simulink model "FormulaElectricSimTool"  (R2015a)
settings: Solver=ode1  StartTime=0.0  StopTime=DriveCycle.Tf  FixedStep=Sim.TimeStep  RelTol=1e-3
undefined symbols (not defined in the file): Battery, Brake, DriveCycle, Driver, g, magnitude, Motor, Sim, Veh
libraries: AMKMotor x4, simulink x3, Battery x1
settings Model: CovSFcnEnable=off  Creator=tbria  LastModifiedBy=tbria
settings DataIOCC: LimitDataPoints=off
settings DebuggingCC: SolverPrmCheckMsg=warning

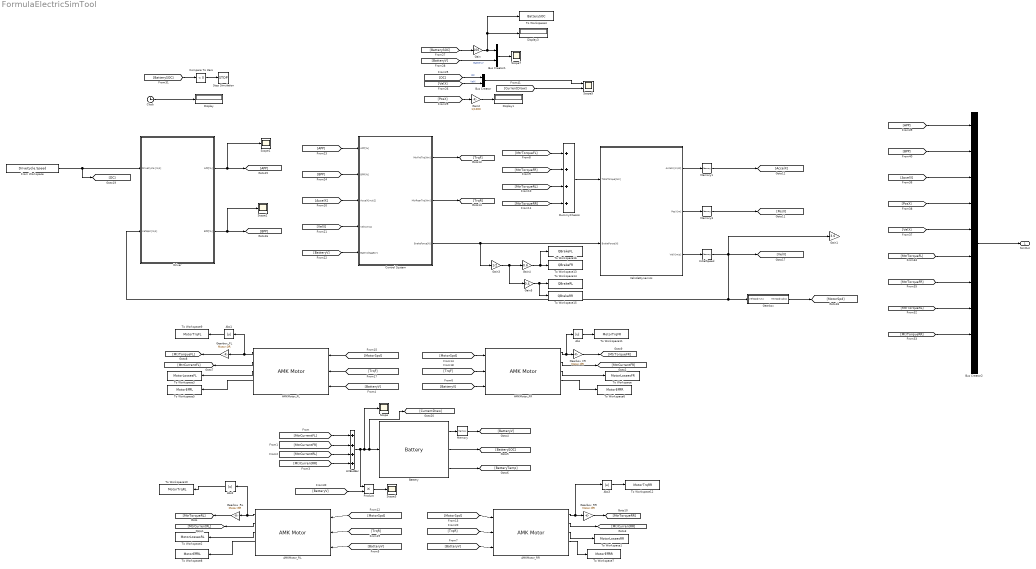
== system FormulaElectricSimTool ==
  AMKMotor_FL : AMKMotor/WheelAssembly/AMK Motor
  AMKMotor_FR : AMKMotor/WheelAssembly/AMK Motor
  AMKMotor_RL : AMKMotor/WheelAssembly/AMK Motor
  AMKMotor_RR : AMKMotor/WheelAssembly/AMK Motor
  Abs{,1..3} (4 alike) : Abs
  Battery : Battery/Battery
  Bus Creator : BusCreator  Inputs=2
  Bus Creator1 : BusCreator  Inputs=2
  Bus Creator2 : BusCreator  Inputs=10
  Clock : Clock
  Compare To Zero : simulink/Logic and Bit Operations/Compare To Zero  relop=<  OutDataTypeStr=boolean
  Control System : Subsystem
  Display : Display
  Display1 : Display
  Display3 : Display
  Driver : Subsystem
  DummyChassis : Sum  Inputs=++++
  From Workspace : FromWorkspace  VariableName=DriveCycle.Speed  SampleTime=0
  Gain : Gain  Gain=100
  Gain1 : Gain  Gain=3.6
  Gain2 : Gain  Gain=1/1000
  Gain3 : Gain  Gain=1/2
  Gain4 : Gain  Gain=0.6
  Gain5 : Gain  Gain=0.4
  Gearbox : Subsystem
  Gearbox_FL : Gain  Gain=Motor.GR
  Gearbox_FR : Gain  Gain=Motor.GR
  Gearbox_RL : Gain  Gain=Motor.GR
  Gearbox_RR : Gain  Gain=Motor.GR
  HVBusBar : Sum  Inputs=4
  InitialSpeed : Memory  X0=DriveCycle.Vi
  Memory : Memory  X0=600
  Memory1 : Memory
  Memory3 : Memory
  Product : Product
  Scope{,1..3,7} (5 alike) : Scope
      Scope2 settings: SaveName=ScopeData2
      Scope3 settings: SaveName=ScopeData3
      Scope7 settings: ShowLegends=on  SaveName=ScopeData7
  Scope5 : Scope  NumInputPorts=2
      settings: ShowLegends=on  YMin=7.5~-5  YMax=37.5~5  SaveName=ScopeData5
  Stop Simulation : Stop
  To Workspace : ToWorkspace  VariableName=MotorLossesFR  SampleTime=-1
      settings: Decimation=3  Save2DSignal=2-D array (concatenate along first dimension)
  To Workspace1 : ToWorkspace  VariableName=MotorLossesRR  SampleTime=-1
      settings: Decimation=3  Save2DSignal=2-D array (concatenate along first dimension)
  To Workspace10 : ToWorkspace  VariableName=MotorTrqRL  SampleTime=-1
      settings: Decimation=3  Save2DSignal=2-D array (concatenate along first dimension)
  To Workspace11 : ToWorkspace  VariableName=MotorTrqFR  SampleTime=-1
      settings: Decimation=3  Save2DSignal=2-D array (concatenate along first dimension)
  To Workspace12 : ToWorkspace  VariableName=MotorTrqRR  SampleTime=-1
      settings: Decimation=3  Save2DSignal=2-D array (concatenate along first dimension)
  To Workspace13 : ToWorkspace  VariableName=QBrakeFR  SampleTime=-1
      settings: Decimation=3  Save2DSignal=2-D array (concatenate along first dimension)
  To Workspace14 : ToWorkspace  VariableName=QBrakeRL  SampleTime=-1
      settings: Decimation=3  Save2DSignal=2-D array (concatenate along first dimension)
  To Workspace15 : ToWorkspace  VariableName=QBrakeRR  SampleTime=-1
      settings: Decimation=3  Save2DSignal=2-D array (concatenate along first dimension)
  To Workspace16 : ToWorkspace  VariableName=QBrakeFL  SampleTime=-1
      settings: Decimation=3  Save2DSignal=2-D array (concatenate along first dimension)
  To Workspace2 : ToWorkspace  VariableName=MotorLossesRL  SampleTime=-1
      settings: Decimation=3  Save2DSignal=2-D array (concatenate along first dimension)
  To Workspace3 : ToWorkspace  VariableName=MotorLossesFL  SampleTime=-1
      settings: Decimation=3  Save2DSignal=2-D array (concatenate along first dimension)
  To Workspace4 : ToWorkspace  VariableName=BatterySOC  SampleTime=-1
      settings: Save2DSignal=2-D array (concatenate along first dimension)
  To Workspace5 : ToWorkspace  VariableName=MotorEffFL  SaveFormat=Timeseries  SampleTime=-1
  To Workspace6 : ToWorkspace  VariableName=MotorEffFR  SaveFormat=Timeseries  SampleTime=-1
  To Workspace7 : ToWorkspace  VariableName=MotorEffRR  SaveFormat=Timeseries  SampleTime=-1
  To Workspace8 : ToWorkspace  VariableName=MotorEffRL  SaveFormat=Timeseries  SampleTime=-1
  To Workspace9 : ToWorkspace  VariableName=MotorTrqFL  SampleTime=-1
      settings: Decimation=3  Save2DSignal=2-D array (concatenate along first dimension)
  VehicleDynamics : Subsystem
  SimOut : Outport
  wires:
  HVBusBar/1 -> Product/1, Scope/1, [CurrentDraw], Battery/1
  [MtrCurrentFL] -> HVBusBar/1
  [MtrCurrentFR] -> HVBusBar/2
  [MtrCurrentRL] -> HVBusBar/3
  [MtrCurrentRR] -> HVBusBar/4
  Battery/1 -> Memory/1
  Battery/2 -> [BatterySOC]
  Battery/3 -> [BatteryTemp]
  [BatteryV] -> AMKMotor_FL/3
  [BatteryV] -> AMKMotor_RL/3
  [BatteryV] -> AMKMotor_RR/3
  AMKMotor_RR/2 -> [MtrCurrentRR]
  AMKMotor_FR/2 -> [MtrCurrentFR]
  AMKMotor_FL/2 -> [MtrCurrentFL]
  AMKMotor_RL/2 -> [MtrCurrentRL]
  [BatteryV] -> AMKMotor_FR/3
  AMKMotor_RL/1 -> Abs2/1, Gearbox_RL/1
  AMKMotor_FL/1 -> Abs1/1, Gearbox_FL/1
  AMKMotor_FR/1 -> Abs/1, Gearbox_FR/1
  AMKMotor_RR/1 -> Abs3/1, Gearbox_RR/1
  Gearbox_RL/1 -> [MtrTorqueRL]
  Gearbox_FL/1 -> [MtrTorqueFL]
  Gearbox_FR/1 -> [MtrTorqueFR]
  Gearbox_RR/1 -> [MtrTorqueRR]
  [MtrTorqueFL] -> DummyChassis/1
  [MtrTorqueFR] -> DummyChassis/2
  [MtrTorqueRL] -> DummyChassis/3
  [MtrTorqueRR] -> DummyChassis/4
  [MotorSpd] -> AMKMotor_RL/1
  [MotorSpd] -> AMKMotor_RR/1
  [MotorSpd] -> AMKMotor_FR/1
  [MotorSpd] -> AMKMotor_FL/1
  [AccelX] -> Control System/3(AccelX[m/s2])
  Control System/2(MtrRearTrq[Nm]) -> [TrqR]
  [TrqF] -> AMKMotor_FL/2
  [TrqF] -> AMKMotor_FR/2
  [TrqR] -> AMKMotor_RL/2
  [TrqR] -> AMKMotor_RR/2
  [VelX] -> Control System/4(VelX[m/s])
  [BatteryV] -> Control System/5(BattVoltage[V])
  Control System/1(MtrFntTrq[Nm]) -> [TrqF]
  Driver/1(APP[%]) -> Scope1/1, [APP]
  Driver/2(BPP[%]) -> Scope2/1, [BPP]
  [APP] -> Control System/1(APP[%])
  [BPP] -> Control System/2(BPP[%])
  DummyChassis/1 -> VehicleDynamics/1(TotalTorque[Nm])
  VehicleDynamics/1(AccelX[m/s2]) -> Memory1/1
  VehicleDynamics/2(PosX[m]) -> Memory3/1
  VehicleDynamics/3(VelX[m/s]) -> InitialSpeed/1
  Gearbox/1(MtrSpd[rad/s]) -> [MotorSpd]
  From Workspace/1 -> [DC], Driver/1(DriveCycle [m/s])
  Clock/1 -> Display/1
  Memory1/1 -> [AccelX]
  Memory/1 -> [BatteryV]
  Memory3/1 -> [PosX]
  InitialSpeed/1 -> Driver/2(VehSpd [m/s]), Gearbox/1(VehSpd[m/s]), Gain1/1, [VelX]
  [DC] -> Bus Creator/1  "DC"
  [VelX] -> Bus Creator/2  "VelX"
  Bus Creator/1 -> Scope5/1
  Control System/3(BrakeForce[N]) -> Gain3/1, VehicleDynamics/2(BrakeForce[N])
  [BatterySOC] -> Gain/1
  [BatteryV] -> Bus Creator1/2  "BatteryV"
  Bus Creator1/1 -> Scope7/1
  Gain/1 -> To Workspace4/1, Display3/1, Bus Creator1/1
  [PosX] -> Gain2/1
  [BatteryV] -> Product/2
  Product/1 -> Scope3/1
  [BatterySOC] -> Compare To Zero/1
  Compare To Zero/1 -> Stop Simulation/1
  AMKMotor_FR/3 -> To Workspace/1
  AMKMotor_RR/3 -> To Workspace1/1
  AMKMotor_RL/3 -> To Workspace2/1
  AMKMotor_FL/3 -> To Workspace3/1
  AMKMotor_FL/4 -> To Workspace5/1
  AMKMotor_FR/4 -> To Workspace6/1
  AMKMotor_RR/4 -> To Workspace7/1
  AMKMotor_RL/4 -> To Workspace8/1
  Abs/1 -> To Workspace11/1
  Abs1/1 -> To Workspace9/1
  Abs2/1 -> To Workspace10/1
  Abs3/1 -> To Workspace12/1
  Bus Creator2/1 -> SimOut/1
  [AccelX] -> Bus Creator2/3
  [APP] -> Bus Creator2/1
  [BPP] -> Bus Creator2/2
  [PosX] -> Bus Creator2/4
  [VelX] -> Bus Creator2/5
  [MtrTorqueFL] -> Bus Creator2/6
  [MtrTorqueFR] -> Bus Creator2/7
  [MtrTorqueRL] -> Bus Creator2/8
  [MtrTorqueRR] -> Bus Creator2/9
  Gain2/1 -> Display1/1
  [CurrentDraw] -> Scope5/2
  Gain3/1 -> Gain5/1, Gain4/1
  Gain4/1 -> To Workspace16/1, To Workspace13/1
  Gain5/1 -> To Workspace15/1, To Workspace14/1

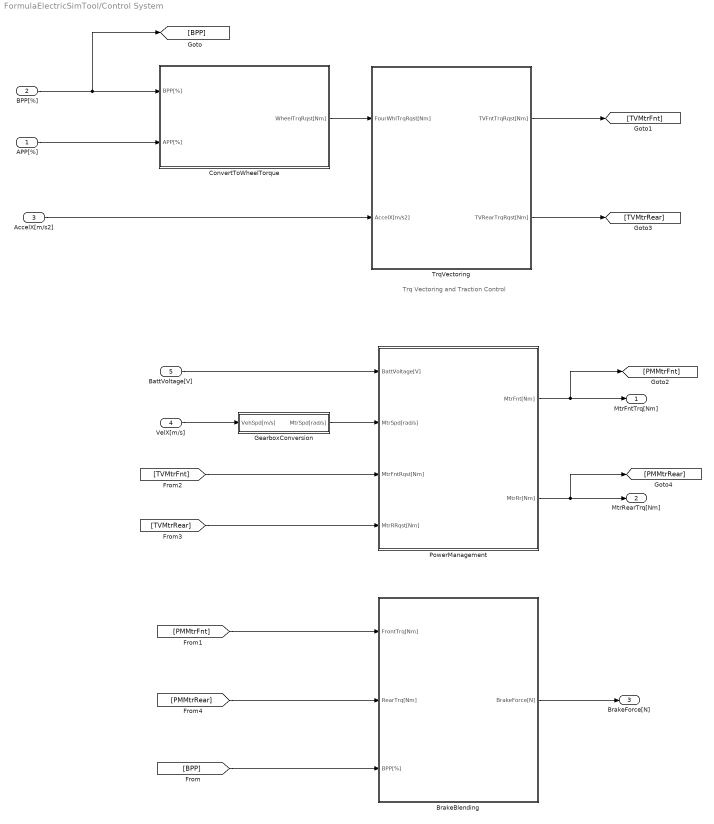
== system FormulaElectricSimTool/Control System ==
  note: Trq Vectoring and Traction Control
  APP[%] : Inport
  BPP[%] : Inport  Port=2
  AccelX[m/s2] : Inport  Port=3
  VelX[m/s] : Inport  Port=4
  BattVoltage[V] : Inport  Port=5
  BrakeBlending : Subsystem
  ConvertToWheelTorque : Subsystem
  GearboxConversion : Subsystem
  PowerManagement : Subsystem
  TrqVectoring : Subsystem
  MtrFntTrq[Nm] : Outport
  MtrRearTrq[Nm] : Outport  Port=2
  BrakeForce[N] : Outport  Port=3
  wires:
  AccelX[m/s2]/1 -> TrqVectoring/2(AccelX[m/s2])
  TrqVectoring/1(TVFntTrqRqst[Nm]) -> [TVMtrFnt]
  TrqVectoring/2(TVRearTrqRqst[Nm]) -> [TVMtrRear]
  BattVoltage[V]/1 -> PowerManagement/1(BattVoltage[V])
  [TVMtrFnt] -> PowerManagement/3(MtrFntRqst[Nm])
  [TVMtrRear] -> PowerManagement/4(MtrRRqst[Nm])
  PowerManagement/1(MtrFnt[Nm]) -> [PMMtrFnt], MtrFntTrq[Nm]/1
  PowerManagement/2(MtrRr[Nm]) -> [PMMtrRear], MtrRearTrq[Nm]/1
  VelX[m/s]/1 -> GearboxConversion/1(VehSpd[m/s])
  GearboxConversion/1(MtrSpd[rad/s]) -> PowerManagement/2(MtrSpd[rad/s])
  ConvertToWheelTorque/1(WheelTrqRqst[Nm]) -> TrqVectoring/1(FourWhlTrqRqst[Nm])
  BrakeBlending/1(BrakeForce[N]) -> BrakeForce[N]/1
  [BPP] -> BrakeBlending/3(BPP[%])
  [PMMtrFnt] -> BrakeBlending/1(FrontTrq[Nm])
  [PMMtrRear] -> BrakeBlending/2(RearTrq[Nm])
  BPP[%]/1 -> [BPP], ConvertToWheelTorque/1(BPP[%])
  APP[%]/1 -> ConvertToWheelTorque/2(APP[%])

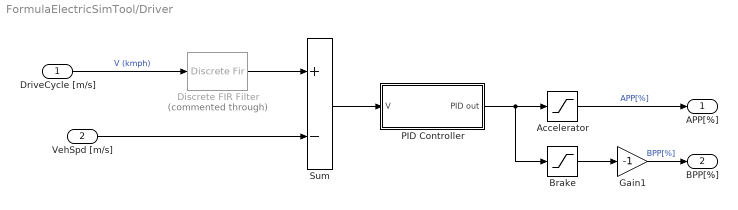
== system FormulaElectricSimTool/Driver ==
  DriveCycle [m/s] : Inport
  VehSpd [m/s] : Inport  Port=2
  Accelerator : Saturate  UpperLimit=100  LowerLimit=0
  Brake : Saturate  UpperLimit=0  LowerLimit=-100
  Discrete FIR Filter : DiscreteFir  Commented=through  Coefficients=[100:-1:0]/sum([100:-1:0])  SampleTime=Sim.TimeStep
  Gain1 : Gain  Gain=-1
  PID Controller : Subsystem
  Sum : Sum  Inputs=+-
  APP[%] : Outport
  BPP[%] : Outport  Port=2
  wires:
  VehSpd [m/s]/1 -> Sum/2
  Sum/1 -> PID Controller/1(V)
  DriveCycle [m/s]/1 -> Discrete FIR Filter/1  "V (kmph)"
  PID Controller/1("PID out ") -> Brake/1, Accelerator/1
  Accelerator/1 -> APP[%]/1  "APP[%]"
  Brake/1 -> Gain1/1
  Gain1/1 -> BPP[%]/1  "BPP[%]"
  Discrete FIR Filter/1 -> Sum/1

== system FormulaElectricSimTool/Gearbox ==
  VehSpd[m/s] : Inport
  MotorGR : Gain  Gain=Motor.GR
  WheelRadius : Gain  Gain=1/(Veh.Whl.r + Veh.Whl.SidewallH)
  MtrSpd[rad/s] : Outport
  wires:
  WheelRadius/1 -> MotorGR/1  "WhlSpd [rad/s]"
  VehSpd[m/s]/1 -> WheelRadius/1
  MotorGR/1 -> MtrSpd[rad/s]/1  "MtrSpd [rad/s]"

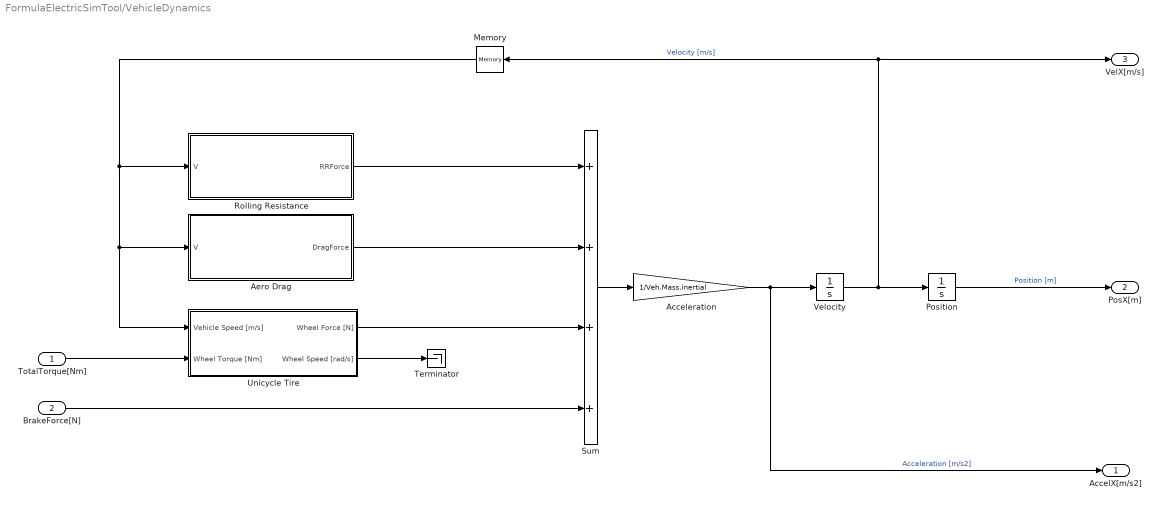
== system FormulaElectricSimTool/VehicleDynamics ==
  TotalTorque[Nm] : Inport
  BrakeForce[N] : Inport  Port=2
  Acceleration : Gain  Gain=1/Veh.Mass.inertial
  Aero Drag : Subsystem
  Memory : Memory
  Position : Integrator
  Rolling Resistance : Subsystem
  Sum : Sum  Inputs=++++
  Terminator : Terminator
  Unicycle Tire : Subsystem
  Velocity : Integrator  InitialCondition=DriveCycle.Vi
  AccelX[m/s2] : Outport
  PosX[m] : Outport  Port=2
  VelX[m/s] : Outport  Port=3
  wires:
  Memory/1 -> Unicycle Tire/1(Vehicle Speed [m/s]), Aero Drag/1(V), Rolling Resistance/1(V)
  Acceleration/1 -> AccelX[m/s2]/1, Velocity/1  "Acceleration [m/s2]"
  TotalTorque[Nm]/1 -> Unicycle Tire/2(Wheel Torque [Nm])
  Rolling Resistance/1(RRForce) -> Sum/1
  Aero Drag/1(DragForce) -> Sum/2
  Sum/1 -> Acceleration/1
  Unicycle Tire/1(Wheel Force [N]) -> Sum/3
  Unicycle Tire/2(Wheel Speed [rad/s]) -> Terminator/1
  Velocity/1 -> VelX[m/s]/1, Memory/1, Position/1  "Velocity [m/s]"
  Position/1 -> PosX[m]/1  "Position [m]"
  BrakeForce[N]/1 -> Sum/4

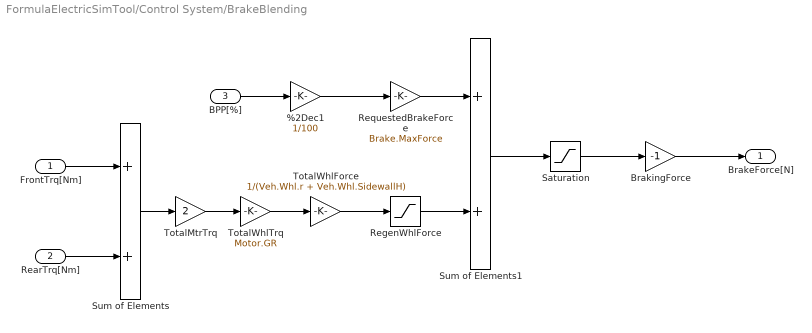
== system FormulaElectricSimTool/Control System/BrakeBlending ==
  FrontTrq[Nm] : Inport
  RearTrq[Nm] : Inport  Port=2
  BPP[%] : Inport  Port=3
  %2Dec1 : Gain  Gain=1/100
  BrakingForce : Gain  Gain=-1
  RegenWhlForce : Saturate  UpperLimit=0  LowerLimit=-inf
  RequestedBrakeForce : Gain  Gain=Brake.MaxForce
  Saturation : Saturate  UpperLimit=inf  LowerLimit=0
  Sum of Elements : Sum  Inputs=2
  Sum of Elements1 : Sum
  TotalMtrTrq : Gain  Gain=2
  TotalWhlForce : Gain  Gain=1/(Veh.Whl.r + Veh.Whl.SidewallH)
  TotalWhlTrq : Gain  Gain=Motor.GR
  BrakeForce[N] : Outport
  wires:
  FrontTrq[Nm]/1 -> Sum of Elements/1
  RearTrq[Nm]/1 -> Sum of Elements/2
  TotalMtrTrq/1 -> TotalWhlTrq/1
  %2Dec1/1 -> RequestedBrakeForce/1
  BPP[%]/1 -> %2Dec1/1
  RequestedBrakeForce/1 -> Sum of Elements1/1
  TotalWhlForce/1 -> RegenWhlForce/1
  Sum of Elements1/1 -> Saturation/1
  Saturation/1 -> BrakingForce/1
  Sum of Elements/1 -> TotalMtrTrq/1
  TotalWhlTrq/1 -> TotalWhlForce/1
  RegenWhlForce/1 -> Sum of Elements1/2
  BrakingForce/1 -> BrakeForce[N]/1

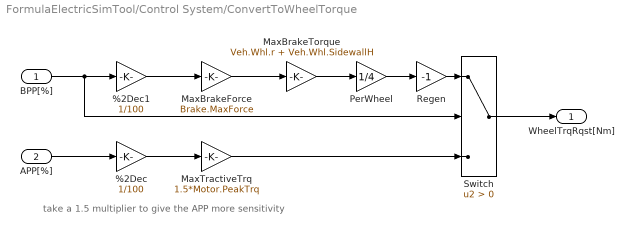
== system FormulaElectricSimTool/Control System/ConvertToWheelTorque ==
  note: take a 1.5 multiplier to give the APP more sensitivity
  BPP[%] : Inport
  APP[%] : Inport  Port=2
  %2Dec : Gain  Gain=1/100
  %2Dec1 : Gain  Gain=1/100
  MaxBrakeForce : Gain  Gain=Brake.MaxForce
  MaxBrakeTorque : Gain  Gain=Veh.Whl.r + Veh.Whl.SidewallH
  "MaxTractiveTrq " : Gain  Gain=1.5*Motor.PeakTrq
  PerWheel : Gain  Gain=1/4
  Regen : Gain  Gain=-1
  Switch : Switch  Criteria=u2 > Threshold
  WheelTrqRqst[Nm] : Outport
  wires:
  PerWheel/1 -> Regen/1
  "MaxTractiveTrq "/1 -> Switch/3
  %2Dec/1 -> "MaxTractiveTrq "/1
  MaxBrakeForce/1 -> MaxBrakeTorque/1
  MaxBrakeTorque/1 -> PerWheel/1
  BPP[%]/1 -> Switch/2, %2Dec1/1
  %2Dec1/1 -> MaxBrakeForce/1
  Switch/1 -> WheelTrqRqst[Nm]/1
  APP[%]/1 -> %2Dec/1
  Regen/1 -> Switch/1

== system FormulaElectricSimTool/Control System/GearboxConversion ==
  VehSpd[m/s] : Inport
  MotorGR : Gain  Gain=Motor.GR
  WheelRadius : Gain  Gain=1/(Veh.Whl.r + Veh.Whl.SidewallH)
  MtrSpd[rad/s] : Outport
  wires:
  WheelRadius/1 -> MotorGR/1  "WhlSpd [rad/s]"
  VehSpd[m/s]/1 -> WheelRadius/1
  MotorGR/1 -> MtrSpd[rad/s]/1  "MtrSpd [rad/s]"

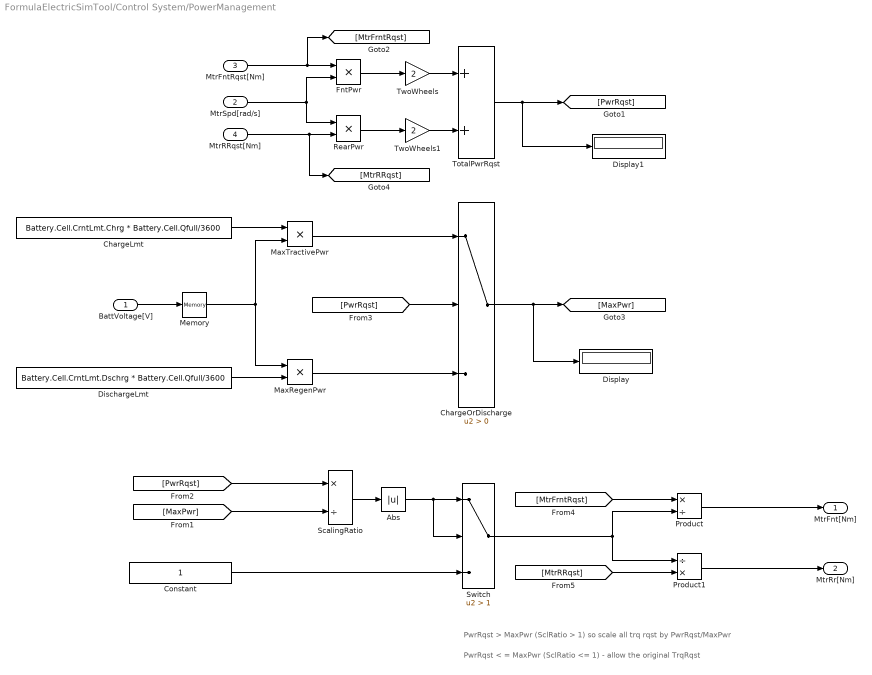
== system FormulaElectricSimTool/Control System/PowerManagement ==
  note: PwrRqst > MaxPwr (SclRatio > 1) so scale all trq rqst by PwrRqst/MaxPwr
  note: PwrRqst < = MaxPwr (SclRatio <= 1) - allow the original TrqRqst
  BattVoltage[V] : Inport
  MtrSpd[rad/s] : Inport  Port=2
  MtrFntRqst[Nm] : Inport  Port=3
  MtrRRqst[Nm] : Inport  Port=4
  Abs : Abs
  ChargeLmt : Constant  Value=Battery.Cell.CrntLmt.Chrg * Battery.Cell.Qfull/3600
  ChargeOrDischarge : Switch  Criteria=u2 > Threshold
  Constant : Constant
  DischargeLmt : Constant  Value=Battery.Cell.CrntLmt.Dschrg * Battery.Cell.Qfull/3600
  Display : Display
  Display1 : Display
  FntPwr : Product
  MaxRegenPwr : Product
  MaxTractivePwr : Product
  Memory : Memory  X0=600
  Product : Product  Inputs=*/
  Product1 : Product  Inputs=/*
  RearPwr : Product
  ScalingRatio : Product  Inputs=*/
  Switch : Switch  Criteria=u2 > Threshold  Threshold=1
  TotalPwrRqst : Sum
  TwoWheels : Gain  Gain=2
  TwoWheels1 : Gain  Gain=2
  MtrFnt[Nm] : Outport
  MtrRr[Nm] : Outport  Port=2
  wires:
  ChargeLmt/1 -> MaxTractivePwr/1
  BattVoltage[V]/1 -> Memory/1
  DischargeLmt/1 -> MaxRegenPwr/2
  MaxTractivePwr/1 -> ChargeOrDischarge/1
  MaxRegenPwr/1 -> ChargeOrDischarge/3
  ChargeOrDischarge/1 -> Display/1, [MaxPwr]
  [MaxPwr] -> ScalingRatio/2
  [PwrRqst] -> ScalingRatio/1
  ScalingRatio/1 -> Abs/1
  Abs/1 -> Switch/1, Switch/2
  MtrSpd[rad/s]/1 -> RearPwr/1, FntPwr/2
  MtrRRqst[Nm]/1 -> [MtrRRqst], RearPwr/2
  FntPwr/1 -> TwoWheels/1
  RearPwr/1 -> TwoWheels1/1
  TwoWheels1/1 -> TotalPwrRqst/2
  TotalPwrRqst/1 -> Display1/1, [PwrRqst]
  TwoWheels/1 -> TotalPwrRqst/1
  [PwrRqst] -> ChargeOrDischarge/2
  MtrFntRqst[Nm]/1 -> [MtrFrntRqst], FntPwr/1
  Switch/1 -> Product/2, Product1/1
  [MtrFrntRqst] -> Product/1
  [MtrRRqst] -> Product1/2
  Product/1 -> MtrFnt[Nm]/1
  Product1/1 -> MtrRr[Nm]/1
  Constant/1 -> Switch/3
  Memory/1 -> MaxTractivePwr/2, MaxRegenPwr/1

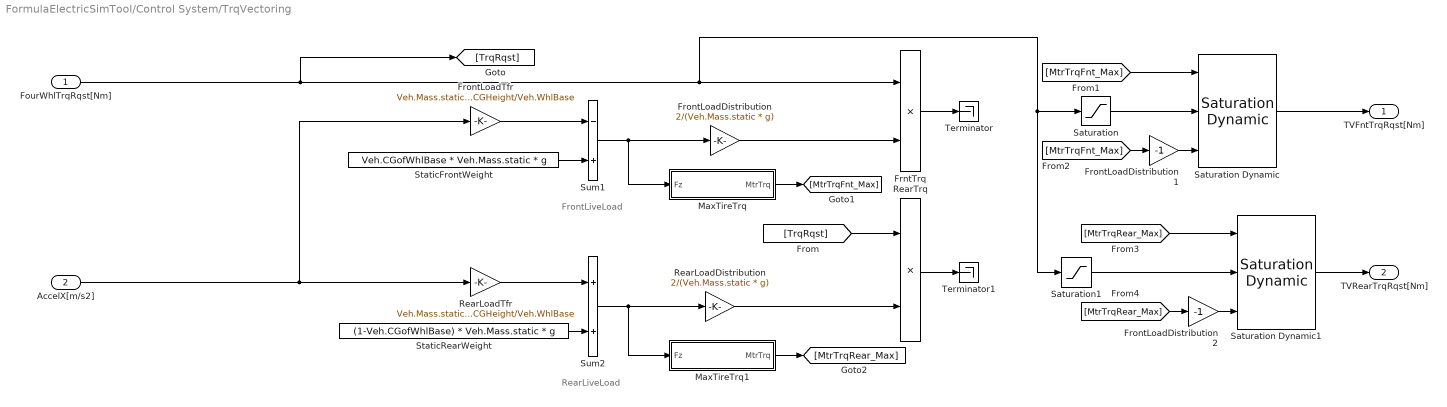
== system FormulaElectricSimTool/Control System/TrqVectoring ==
  note: RearLiveLoad
  note: FrontLiveLoad
  FourWhlTrqRqst[Nm] : Inport
  AccelX[m/s2] : Inport  Port=2
  FrntTrq : Product
  FrontLoadDistribution : Gain  Gain=2/(Veh.Mass.static * g)
  FrontLoadDistribution1 : Gain  Gain=-1
  FrontLoadDistribution2 : Gain  Gain=-1
  FrontLoadTfr : Gain  Gain=Veh.Mass.static*Veh.CGHeight/Veh.WhlBase
  MaxTireTrq : Subsystem
  MaxTireTrq1 : Subsystem
  RearLoadDistribution : Gain  Gain=2/(Veh.Mass.static * g)
  RearLoadTfr : Gain  Gain=Veh.Mass.static*Veh.CGHeight/Veh.WhlBase
  RearTrq : Product
  Saturation : Saturate  UpperLimit=Motor.PeakTrq  LowerLimit=-Motor.PeakTrq
  Saturation Dynamic : simulink/Discontinuities/Saturation Dynamic  OutMin=[]  OutMax=[]  OutDataTypeStr=Inherit: Same as second input  OutDataType=fixdt(1, 16)  OutScaling=2^-10  DoSatur=off
  Saturation Dynamic1 : simulink/Discontinuities/Saturation Dynamic  OutMin=[]  OutMax=[]  OutDataTypeStr=Inherit: Same as second input  OutDataType=fixdt(1, 16)  OutScaling=2^-10  DoSatur=off
  Saturation1 : Saturate  UpperLimit=Motor.PeakTrq  LowerLimit=-Motor.PeakTrq
  StaticFrontWeight : Constant  Value=Veh.CGofWhlBase * Veh.Mass.static * g
  StaticRearWeight : Constant  Value=(1-Veh.CGofWhlBase) * Veh.Mass.static * g
  Sum1 : Sum  Inputs=-+
  Sum2 : Sum
  Terminator : Terminator
  Terminator1 : Terminator
  TVFntTrqRqst[Nm] : Outport
  TVRearTrqRqst[Nm] : Outport  Port=2
  wires:
  AccelX[m/s2]/1 -> RearLoadTfr/1, FrontLoadTfr/1
  Sum1/1 -> MaxTireTrq/1(Fz), FrontLoadDistribution/1
  FrontLoadTfr/1 -> Sum1/1
  StaticFrontWeight/1 -> Sum1/2
  RearLoadTfr/1 -> Sum2/1
  Sum2/1 -> MaxTireTrq1/1(Fz), RearLoadDistribution/1
  StaticRearWeight/1 -> Sum2/2
  FrontLoadDistribution/1 -> FrntTrq/2
  RearLoadDistribution/1 -> RearTrq/2
  [TrqRqst] -> RearTrq/1
  FourWhlTrqRqst[Nm]/1 -> [TrqRqst], Saturation1/1, Saturation/1, FrntTrq/1
  Saturation/1 -> Saturation Dynamic/2
  Saturation Dynamic/1 -> TVFntTrqRqst[Nm]/1
  MaxTireTrq/1(MtrTrq) -> [MtrTrqFnt_Max]
  MaxTireTrq1/1(MtrTrq) -> [MtrTrqRear_Max]
  [MtrTrqFnt_Max] -> Saturation Dynamic/1
  [MtrTrqFnt_Max] -> FrontLoadDistribution1/1
  FrontLoadDistribution1/1 -> Saturation Dynamic/3
  Saturation1/1 -> Saturation Dynamic1/2
  Saturation Dynamic1/1 -> TVRearTrqRqst[Nm]/1
  [MtrTrqRear_Max] -> Saturation Dynamic1/1
  [MtrTrqRear_Max] -> FrontLoadDistribution2/1
  FrontLoadDistribution2/1 -> Saturation Dynamic1/3
  FrntTrq/1 -> Terminator/1
  RearTrq/1 -> Terminator1/1

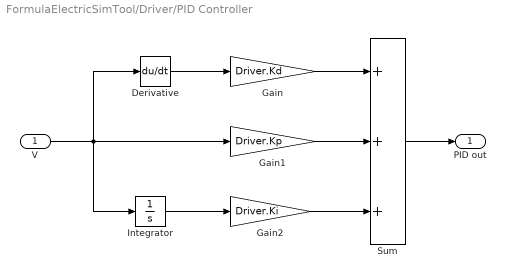
== system FormulaElectricSimTool/Driver/PID Controller ==
  V : Inport
  Derivative : Derivative
  Gain : Gain  Gain=Driver.Kd
  Gain1 : Gain  Gain=Driver.Kp
  Gain2 : Gain  Gain=Driver.Ki
  Integrator : Integrator
  Sum : Sum  Inputs=+++
  "PID out " : Outport
  wires:
  Integrator/1 -> Gain2/1
  V/1 -> Integrator/1, Derivative/1, Gain1/1
  Gain/1 -> Sum/1
  Gain1/1 -> Sum/2
  Gain2/1 -> Sum/3
  Sum/1 -> "PID out "/1
  Derivative/1 -> Gain/1

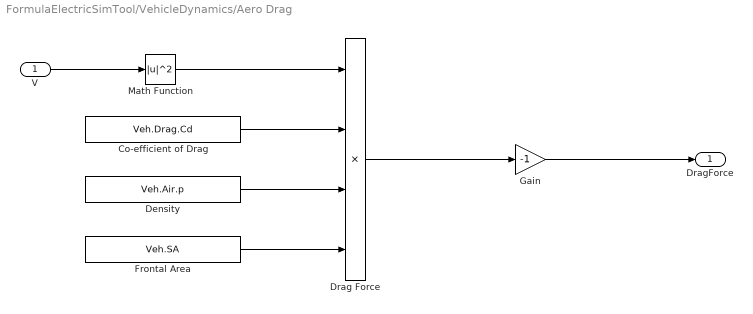
== system FormulaElectricSimTool/VehicleDynamics/Aero Drag ==
  V : Inport
  Co-efficient of Drag : Constant  Value=Veh.Drag.Cd
  Density : Constant  Value=Veh.Air.p
  Drag Force : Product  Inputs=****
  Frontal Area : Constant  Value=Veh.SA
  Gain : Gain  Gain=-1
  Math Function : Math  Operator=magnitude^2  SaturateOnIntegerOverflow=on
  DragForce : Outport
  wires:
  Co-efficient of Drag/1 -> Drag Force/2
  Drag Force/1 -> Gain/1
  V/1 -> Math Function/1
  Math Function/1 -> Drag Force/1
  Density/1 -> Drag Force/3
  Frontal Area/1 -> Drag Force/4
  Gain/1 -> DragForce/1

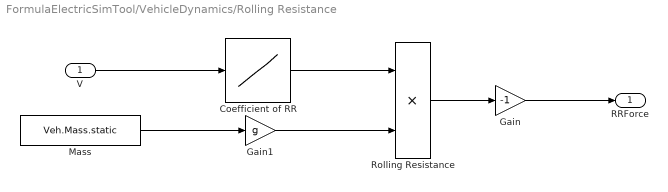
== system FormulaElectricSimTool/VehicleDynamics/Rolling Resistance ==
  V : Inport
  Coefficient of RR : Lookup_n-D  NumberOfTableDimensions=1  BreakpointsForDimension1=Veh.Tires.rr.Spd  BreakpointsForDimension2=Motor.Efficiency.Spd  Table=Veh.Tires.rr.rr  InternalRulePriority=Speed  RndMeth=Simplest  InputSameDT=on
  Gain : Gain  Gain=-1
  Gain1 : Gain  Gain=g
  Mass : Constant  Value=Veh.Mass.static
  Rolling Resistance : Product
  RRForce : Outport
  wires:
  Rolling Resistance/1 -> Gain/1
  V/1 -> Coefficient of RR/1
  Gain/1 -> RRForce/1
  Coefficient of RR/1 -> Rolling Resistance/1
  Mass/1 -> Gain1/1
  Gain1/1 -> Rolling Resistance/2

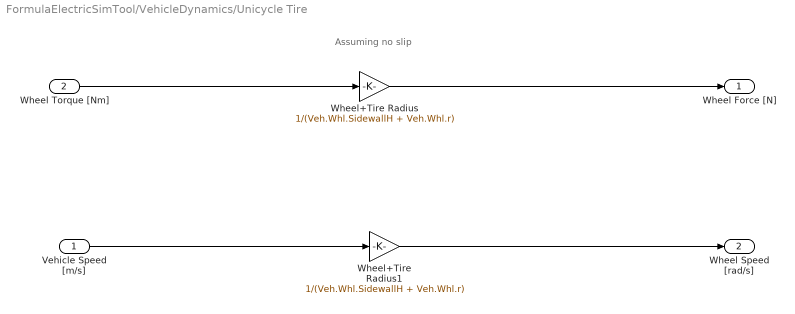
== system FormulaElectricSimTool/VehicleDynamics/Unicycle Tire ==
  note: Assuming no slip
  Vehicle Speed [m/s] : Inport
  Wheel Torque [Nm] : Inport  Port=2
  Wheel+Tire Radius : Gain  Gain=1/(Veh.Whl.SidewallH + Veh.Whl.r)
  Wheel+Tire Radius1 : Gain  Gain=1/(Veh.Whl.SidewallH + Veh.Whl.r)
  Wheel Force [N] : Outport
  Wheel Speed [rad/s] : Outport  Port=2
  wires:
  Wheel Torque [Nm]/1 -> Wheel+Tire Radius/1
  Wheel+Tire Radius/1 -> Wheel Force [N]/1
  Vehicle Speed [m/s]/1 -> Wheel+Tire Radius1/1
  Wheel+Tire Radius1/1 -> Wheel Speed [rad/s]/1

== system FormulaElectricSimTool/Control System/TrqVectoring/MaxTireTrq ==
  Fz : Inport
  MaxMtrTorque : Gain  Gain=1/Motor.GR
  MaxTireForce : Gain  Gain=Veh.Tires.Ks
  MaxWhlTorque : Gain  Gain=Veh.Whl.r + Veh.Whl.SidewallH
  SplitAxle : Gain  Gain=1/2
  MtrTrq : Outport
  wires:
  MaxTireForce/1 -> MaxWhlTorque/1
  Fz/1 -> SplitAxle/1
  MaxWhlTorque/1 -> MaxMtrTorque/1
  SplitAxle/1 -> MaxTireForce/1
  MaxMtrTorque/1 -> MtrTrq/1

== system FormulaElectricSimTool/Control System/TrqVectoring/MaxTireTrq1 ==
  Fz : Inport
  MaxMtrTorque : Gain  Gain=1/Motor.GR
  MaxTireForce : Gain  Gain=Veh.Tires.Ks
  MaxWhlTorque : Gain  Gain=Veh.Whl.r + Veh.Whl.SidewallH
  SplitAxle : Gain  Gain=1/2
  MtrTrq : Outport
  wires:
  MaxTireForce/1 -> MaxWhlTorque/1
  Fz/1 -> SplitAxle/1
  MaxWhlTorque/1 -> MaxMtrTorque/1
  SplitAxle/1 -> MaxTireForce/1
  MaxMtrTorque/1 -> MtrTrq/1
